simulink model "Ex5"  (R2021a)
settings: Solver=VariableStepAuto  StartTime=0.0  StopTime=10.0  RelTol=1e-3
libraries: dspstat3 x1
settings Model: Creator=gferr  LastModifiedBy=gferr

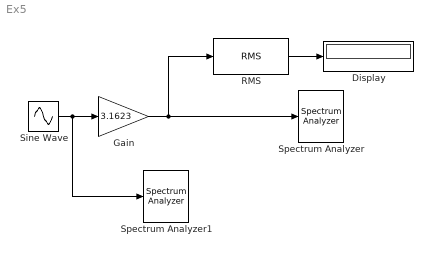
== system Ex5 ==
  Display : Display
  Gain : Gain  Gain=3.1623
  RMS : dspstat3/RMS  run=off  directionMode=Each column  dimension=1  InputProcessing=Columns as channels (frame based)  reset_popup=None
  Sine Wave : Sin  Amplitude=0.5  Frequency=3.5e9  SampleTime=1e-10
  Spectrum Analyzer : SpectrumAnalyzer
  Spectrum Analyzer1 : SpectrumAnalyzer
  wires:
  Sine Wave/1 -> Spectrum Analyzer1/1, Gain/1
  Gain/1 -> RMS/1, Spectrum Analyzer/1
  RMS/1 -> Display/1
